simulink model "model"  (R2014a)
(part 8 of 8)

  _CN_287115458_300000_CN_287115460_300000/RConn3 -- T_287115460__/LConn3 -- bus157/LConn1
  _CN_287115458_300000_CN_355844786_300000/RConn1 -- T_355844786_300000_Hof_transformator/LConn1 -- _CN_355844786_300000_CN_51854396_300000/LConn1
  _CN_287115458_300000_CN_355844786_300000/RConn2 -- T_355844786_300000_Hof_transformator/LConn2 -- _CN_355844786_300000_CN_51854396_300000/LConn2
  _CN_287115458_300000_CN_355844786_300000/RConn3 -- T_355844786_300000_Hof_transformator/LConn3 -- _CN_355844786_300000_CN_51854396_300000/LConn3 -- bus158/LConn1
  Førre_Saurdal_CN_285935887_300000_CN_285915728_300000/RConn1 -- T_285935887__Saurdal_transformatorstasjon/RConn1 -- L_285935887/LConn1
  Førre_Saurdal_CN_285935887_300000_CN_285915728_300000/RConn2 -- T_285935887__Saurdal_transformatorstasjon/RConn2 -- L_285935887/LConn2
  Førre_Saurdal_CN_285935887_300000_CN_285915728_300000/RConn3 -- T_285935887__Saurdal_transformatorstasjon/RConn3 -- L_285935887/LConn3 -- bus159/LConn1
  _CN_355844786_300000_CN_51854396_300000/RConn1 -- T_51854396_420000;300000;132000_Tveiten/RConn1 -- _CN_206538656_300000_CN_51854396_300000/LConn1
  _CN_355844786_300000_CN_51854396_300000/RConn2 -- T_51854396_420000;300000;132000_Tveiten/RConn2 -- _CN_206538656_300000_CN_51854396_300000/LConn2
  _CN_355844786_300000_CN_51854396_300000/RConn3 -- T_51854396_420000;300000;132000_Tveiten/RConn3 -- _CN_206538656_300000_CN_51854396_300000/LConn3 -- bus160/LConn1
  Feda_Åna_Sira_CN_284275993_300000_CN_174418125_300000/LConn1 -- T_284275993_300000_/LConn1 -- Åna_Sira_Kjelland_CN_284275993_300000_CN_124861857_300000/LConn1
  Feda_Åna_Sira_CN_284275993_300000_CN_174418125_300000/LConn2 -- T_284275993_300000_/LConn2 -- Åna_Sira_Kjelland_CN_284275993_300000_CN_124861857_300000/LConn2
  Feda_Åna_Sira_CN_284275993_300000_CN_174418125_300000/LConn3 -- T_284275993_300000_/LConn3 -- Åna_Sira_Kjelland_CN_284275993_300000_CN_124861857_300000/LConn3 -- bus161/LConn1
  Feda_Åna_Sira_CN_284275993_300000_CN_174418125_300000/RConn1 -- T_174418125_300000_Feda_trafostasjon/LConn1 -- Feda_Vennesla_CN_287687994_300000_CN_174418125_300000/LConn1 -- _CN_296076234_300000_CN_174418125_300000/LConn1 -- _CN_174418125_300000_CN_174418126_300000/LConn1 -- Tonstad_Feda_CN_285825051_300000_CN_174418125_300000/RConn1
  Feda_Åna_Sira_CN_284275993_300000_CN_174418125_300000/RConn2 -- T_174418125_300000_Feda_trafostasjon/LConn2 -- Feda_Vennesla_CN_287687994_300000_CN_174418125_300000/LConn2 -- _CN_296076234_300000_CN_174418125_300000/LConn2 -- _CN_174418125_300000_CN_174418126_300000/LConn2 -- Tonstad_Feda_CN_285825051_300000_CN_174418125_300000/RConn2
  Feda_Åna_Sira_CN_284275993_300000_CN_174418125_300000/RConn3 -- T_174418125_300000_Feda_trafostasjon/LConn3 -- Feda_Vennesla_CN_287687994_300000_CN_174418125_300000/LConn3 -- _CN_296076234_300000_CN_174418125_300000/LConn3 -- _CN_174418125_300000_CN_174418126_300000/LConn3 -- bus162/LConn1 -- Tonstad_Feda_CN_285825051_300000_CN_174418125_300000/RConn3
  Åna_Sira_Kjelland_CN_284275993_300000_CN_124861857_300000/RConn1 -- T_124861857__Kjelland_transformatorstasjon/LConn1 -- Kjelland_Stokkeland_CN_124861857_300000_CN_88147266_300000/RConn1
  Åna_Sira_Kjelland_CN_284275993_300000_CN_124861857_300000/RConn2 -- T_124861857__Kjelland_transformatorstasjon/LConn2 -- Kjelland_Stokkeland_CN_124861857_300000_CN_88147266_300000/RConn2
  Åna_Sira_Kjelland_CN_284275993_300000_CN_124861857_300000/RConn3 -- T_124861857__Kjelland_transformatorstasjon/LConn3 -- Kjelland_Stokkeland_CN_124861857_300000_CN_88147266_300000/RConn3 -- bus163/LConn1
  Solhom_Tonstad_CN_285825051_300000_CN_295295263_300000/RConn1 -- T_295295263__/LConn1 -- Arendal_Solhom_CN_295295263_300000_CN_297392932_300000/LConn1
  Solhom_Tonstad_CN_285825051_300000_CN_295295263_300000/RConn2 -- T_295295263__/LConn2 -- Arendal_Solhom_CN_295295263_300000_CN_297392932_300000/LConn2
  Solhom_Tonstad_CN_285825051_300000_CN_295295263_300000/RConn3 -- T_295295263__/LConn3 -- Arendal_Solhom_CN_295295263_300000_CN_297392932_300000/LConn3 -- bus164/LConn1
  Arendal_Solhom_CN_295295263_300000_CN_297392932_300000/RConn1 -- T_297392932__Arendal_transformator/LConn1 -- Arendal_Vennesla_CN_287687994_300000_CN_297392932_300000/LConn1 -- _CN_297392932_300000_CN_358915801_300000/LConn1
  Arendal_Solhom_CN_295295263_300000_CN_297392932_300000/RConn2 -- T_297392932__Arendal_transformator/LConn2 -- Arendal_Vennesla_CN_287687994_300000_CN_297392932_300000/LConn2 -- _CN_297392932_300000_CN_358915801_300000/LConn2
  Arendal_Solhom_CN_295295263_300000_CN_297392932_300000/RConn3 -- T_297392932__Arendal_transformator/LConn3 -- Arendal_Vennesla_CN_287687994_300000_CN_297392932_300000/LConn3 -- _CN_297392932_300000_CN_358915801_300000/LConn3 -- bus165/LConn1
  Eidanger_Rød_CN_206538656_300000_CN_100648754_300000/LConn1 -- T_206538656_420000;300000;132000_Rød_transformatorstasjon/RConn1 -- _CN_206538656_300000_CN_51854396_300000/RConn1
  Eidanger_Rød_CN_206538656_300000_CN_100648754_300000/LConn2 -- T_206538656_420000;300000;132000_Rød_transformatorstasjon/RConn2 -- _CN_206538656_300000_CN_51854396_300000/RConn2
  Eidanger_Rød_CN_206538656_300000_CN_100648754_300000/LConn3 -- T_206538656_420000;300000;132000_Rød_transformatorstasjon/RConn3 -- _CN_206538656_300000_CN_51854396_300000/RConn3 -- bus166/LConn1
  Eidanger_Rød_CN_206538656_300000_CN_100648754_300000/RConn1 -- T_100648754_300000;132000_/LConn1 -- Bamble_Porsgrunn_CN_100648754_300000_CN_206628449_300000/LConn1
  Eidanger_Rød_CN_206538656_300000_CN_100648754_300000/RConn2 -- T_100648754_300000;132000_/LConn2 -- Bamble_Porsgrunn_CN_100648754_300000_CN_206628449_300000/LConn2
  Eidanger_Rød_CN_206538656_300000_CN_100648754_300000/RConn3 -- T_100648754_300000;132000_/LConn3 -- Bamble_Porsgrunn_CN_100648754_300000_CN_206628449_300000/LConn3 -- bus167/LConn1
  Rjukan_Songa_CN_288685602_300000_CN_288812256_300000/RConn1 -- T_288812256__Songa_kraftverk/LConn1 -- Kvilldal_Songa_CN_288812256_300000_CN_214181609_300000/LConn1 -- Songa_Vinje_CN_285750826_300000_CN_288812256_300000/LConn1
  Rjukan_Songa_CN_288685602_300000_CN_288812256_300000/RConn2 -- T_288812256__Songa_kraftverk/LConn2 -- Kvilldal_Songa_CN_288812256_300000_CN_214181609_300000/LConn2 -- Songa_Vinje_CN_285750826_300000_CN_288812256_300000/LConn2
  Rjukan_Songa_CN_288685602_300000_CN_288812256_300000/RConn3 -- T_288812256__Songa_kraftverk/LConn3 -- Kvilldal_Songa_CN_288812256_300000_CN_214181609_300000/LConn3 -- bus168/LConn1 -- Songa_Vinje_CN_285750826_300000_CN_288812256_300000/LConn3
  T_265770276__/LConn1 -- _CN_265770276_300000_CN_297388897_300000/LConn1
  T_265770276__/LConn2 -- _CN_265770276_300000_CN_297388897_300000/LConn2
  _CN_265770276_300000_CN_297388897_300000/LConn3 -- T_265770276__/LConn3 -- bus169/LConn1
  T_297388897_300000_Fåberg_trafostasjon/LConn1 -- _CN_265770276_300000_CN_297388897_300000/RConn1
  T_297388897_300000_Fåberg_trafostasjon/LConn2 -- _CN_265770276_300000_CN_297388897_300000/RConn2
  _CN_265770276_300000_CN_297388897_300000/RConn3 -- T_297388897_300000_Fåberg_trafostasjon/LConn3 -- bus170/LConn1
  T_290373414_300000;132000_/LConn1 -- _CN_290373414_300000_CN_290390502_300000/LConn1
  T_290373414_300000;132000_/LConn2 -- _CN_290373414_300000_CN_290390502_300000/LConn2
  _CN_290373414_300000_CN_290390502_300000/LConn3 -- T_290373414_300000;132000_/LConn3 -- bus171/LConn1
  _CN_290373414_300000_CN_290390502_300000/RConn1 -- T_290390502_300000_/LConn1 -- _CN_330825503_300000_CN_290390502_300000/LConn1
  _CN_290373414_300000_CN_290390502_300000/RConn2 -- T_290390502_300000_/LConn2 -- _CN_330825503_300000_CN_290390502_300000/LConn2
  _CN_290373414_300000_CN_290390502_300000/RConn3 -- T_290390502_300000_/LConn3 -- _CN_330825503_300000_CN_290390502_300000/LConn3 -- bus172/LConn1
  T_288810920__/LConn1 -- Nesflaten_Rjukan_CN_288810920_300000_CN_430780474_300000/LConn1
  T_288810920__/LConn2 -- Nesflaten_Rjukan_CN_288810920_300000_CN_430780474_300000/LConn2
  Nesflaten_Rjukan_CN_288810920_300000_CN_430780474_300000/LConn3 -- T_288810920__/LConn3 -- bus173/LConn1
  T_430780474__/LConn1 -- Nesflaten_Rjukan_CN_288810920_300000_CN_430780474_300000/RConn1
  T_430780474__/LConn2 -- Nesflaten_Rjukan_CN_288810920_300000_CN_430780474_300000/RConn2
  Nesflaten_Rjukan_CN_288810920_300000_CN_430780474_300000/RConn3 -- T_430780474__/LConn3 -- bus174/LConn1
  T_285750826__Vinje_kraftverk/LConn1 -- Songa_Vinje_CN_285750826_300000_CN_288812256_300000/RConn1
  T_285750826__Vinje_kraftverk/LConn2 -- Songa_Vinje_CN_285750826_300000_CN_288812256_300000/RConn2
  Songa_Vinje_CN_285750826_300000_CN_288812256_300000/RConn3 -- T_285750826__Vinje_kraftverk/LConn3 -- bus175/LConn1
  T_109810733_300000;132000_Smestad_trafostasjon/LConn1 -- _CN_46873771_300000_CN_109810733_300000/RConn1
  T_109810733_300000;132000_Smestad_trafostasjon/LConn2 -- _CN_46873771_300000_CN_109810733_300000/RConn2
  _CN_46873771_300000_CN_109810733_300000/RConn3 -- T_109810733_300000;132000_Smestad_trafostasjon/LConn3 -- bus176/LConn1
  T_229396655__/LConn1 -- _CN_229396655_300000_CN_333991713_300000/LConn1
  T_229396655__/LConn2 -- _CN_229396655_300000_CN_333991713_300000/LConn2
  _CN_229396655_300000_CN_333991713_300000/LConn3 -- T_229396655__/LConn3 -- bus177/LConn1
  _CN_229396655_300000_CN_333991713_300000/RConn1 -- T_333991713__Fana_transformatorstasjon/LConn1 -- Fana_Samnanger_CN_333991713_300000_CN_350332649_300000/LConn1 -- _CN_333991713_300000_CN_259135596_300000/LConn1
  _CN_229396655_300000_CN_333991713_300000/RConn2 -- T_333991713__Fana_transformatorstasjon/LConn2 -- Fana_Samnanger_CN_333991713_300000_CN_350332649_300000/LConn2 -- _CN_333991713_300000_CN_259135596_300000/LConn2
  _CN_229396655_300000_CN_333991713_300000/RConn3 -- T_333991713__Fana_transformatorstasjon/LConn3 -- Fana_Samnanger_CN_333991713_300000_CN_350332649_300000/LConn3 -- _CN_333991713_300000_CN_259135596_300000/LConn3 -- bus178/LConn1
  T_350332649__Samnanger/LConn1 -- Fana_Samnanger_CN_333991713_300000_CN_350332649_300000/RConn1
  T_350332649__Samnanger/LConn2 -- Fana_Samnanger_CN_333991713_300000_CN_350332649_300000/RConn2
  Fana_Samnanger_CN_333991713_300000_CN_350332649_300000/RConn3 -- T_350332649__Samnanger/LConn3 -- bus179/LConn1
  T_259135596__/LConn1 -- _CN_333991713_300000_CN_259135596_300000/RConn1
  T_259135596__/LConn2 -- _CN_333991713_300000_CN_259135596_300000/RConn2
  _CN_333991713_300000_CN_259135596_300000/RConn3 -- T_259135596__/LConn3 -- bus180/LConn1
  Bamble_Porsgrunn_CN_100648754_300000_CN_206628449_300000/RConn1 -- T_206628449__Bamble/RConn1 -- L_206628449/LConn1
  Bamble_Porsgrunn_CN_100648754_300000_CN_206628449_300000/RConn2 -- T_206628449__Bamble/RConn2 -- L_206628449/LConn2
  Bamble_Porsgrunn_CN_100648754_300000_CN_206628449_300000/RConn3 -- T_206628449__Bamble/RConn3 -- L_206628449/LConn3 -- bus181/LConn1
  T_114336709_300000;132000_Vang_trafostasjon/LConn1 -- Minne_Brenneriroa_CN_120279477_300000_CN_114336709_300000/RConn1
  T_114336709_300000;132000_Vang_trafostasjon/LConn2 -- Minne_Brenneriroa_CN_120279477_300000_CN_114336709_300000/RConn2
  Minne_Brenneriroa_CN_120279477_300000_CN_114336709_300000/RConn3 -- T_114336709_300000;132000_Vang_trafostasjon/LConn3 -- bus182/LConn1
  Førre_Hylen_CN_285915728_300000_CN_289304147_300000/RConn1 -- T_289304147__/LConn1 -- Sauda_Hylen_CN_289304147_300000_CN_285805418_300000/RConn1
  Førre_Hylen_CN_285915728_300000_CN_289304147_300000/RConn2 -- T_289304147__/LConn2 -- Sauda_Hylen_CN_289304147_300000_CN_285805418_300000/RConn2
  Førre_Hylen_CN_285915728_300000_CN_289304147_300000/RConn3 -- T_289304147__/LConn3 -- Sauda_Hylen_CN_289304147_300000_CN_285805418_300000/RConn3 -- bus183/LConn1
  Arendal_Vennesla_CN_287687994_300000_CN_297392932_300000/RConn1 -- T_287687994_420000;300000_/RConn1 -- Feda_Vennesla_CN_287687994_300000_CN_174418125_300000/RConn1
  Arendal_Vennesla_CN_287687994_300000_CN_297392932_300000/RConn2 -- T_287687994_420000;300000_/RConn2 -- Feda_Vennesla_CN_287687994_300000_CN_174418125_300000/RConn2
  Arendal_Vennesla_CN_287687994_300000_CN_297392932_300000/RConn3 -- T_287687994_420000;300000_/RConn3 -- Feda_Vennesla_CN_287687994_300000_CN_174418125_300000/RConn3 -- bus184/LConn1
  T_330825503_300000;132000_/LConn1 -- _CN_330825503_300000_CN_290390502_300000/RConn1
  T_330825503_300000;132000_/LConn2 -- _CN_330825503_300000_CN_290390502_300000/RConn2
  _CN_330825503_300000_CN_290390502_300000/RConn3 -- T_330825503_300000;132000_/LConn3 -- bus185/LConn1
  _CN_296076234_300000_CN_296076235_300000/LConn1 -- T_296076234_300000_/LConn1 -- _CN_296076234_300000_CN_174418125_300000/RConn1
  _CN_296076234_300000_CN_296076235_300000/LConn2 -- T_296076234_300000_/LConn2 -- _CN_296076234_300000_CN_174418125_300000/RConn2
  _CN_296076234_300000_CN_296076235_300000/LConn3 -- T_296076234_300000_/LConn3 -- _CN_296076234_300000_CN_174418125_300000/RConn3 -- bus186/LConn1
  T_296076235_300000;132000_/LConn1 -- _CN_296076234_300000_CN_296076235_300000/RConn1
  T_296076235_300000;132000_/LConn2 -- _CN_296076234_300000_CN_296076235_300000/RConn2
  _CN_296076234_300000_CN_296076235_300000/RConn3 -- T_296076235_300000;132000_/LConn3 -- bus187/LConn1
  T_174418126_300000_Feda_static_inverter_plant/LConn1 -- _CN_174418125_300000_CN_174418126_300000/RConn1
  T_174418126_300000_Feda_static_inverter_plant/LConn2 -- _CN_174418125_300000_CN_174418126_300000/RConn2
  _CN_174418125_300000_CN_174418126_300000/RConn3 -- T_174418126_300000_Feda_static_inverter_plant/LConn3 -- bus188/LConn1
  T_400655825_300000;132000_/LConn1 -- _CN_400655825_300000_CN_201483501_300000/LConn1
  T_400655825_300000;132000_/LConn2 -- _CN_400655825_300000_CN_201483501_300000/LConn2
  _CN_400655825_300000_CN_201483501_300000/LConn3 -- T_400655825_300000;132000_/LConn3 -- bus189/LConn1
  _CN_400655825_300000_CN_201483501_300000/RConn1 -- T_201483501_420000;300000;132000_/RConn1 -- L_201483501/LConn1
  _CN_400655825_300000_CN_201483501_300000/RConn2 -- T_201483501_420000;300000;132000_/RConn2 -- L_201483501/LConn2
  _CN_400655825_300000_CN_201483501_300000/RConn3 -- T_201483501_420000;300000;132000_/RConn3 -- L_201483501/LConn3 -- bus190/LConn1
  T_289304185__/LConn1 -- _CN_289304185_300000_CN_285805418_300000/RConn1
  T_289304185__/LConn2 -- _CN_289304185_300000_CN_285805418_300000/RConn2
  _CN_289304185_300000_CN_285805418_300000/RConn3 -- T_289304185__/LConn3 -- bus191/LConn1
  _CN_297392932_300000_CN_358915801_300000/RConn1 -- T_358915801_420000_/RConn1 -- L_358915801/LConn1
  _CN_297392932_300000_CN_358915801_300000/RConn2 -- T_358915801_420000_/RConn2 -- L_358915801/LConn2
  _CN_297392932_300000_CN_358915801_300000/RConn3 -- T_358915801_420000_/RConn3 -- L_358915801/LConn3 -- bus192/LConn1
  G_71356608_Roskrepp_kraftverk/RConn1 -- Roskrepp_Duge_CN_261717967_300000_CN_71356608_300000/RConn1
  G_71356608_Roskrepp_kraftverk/RConn2 -- Roskrepp_Duge_CN_261717967_300000_CN_71356608_300000/RConn2
  Roskrepp_Duge_CN_261717967_300000_CN_71356608_300000/RConn3 -- G_71356608_Roskrepp_kraftverk/RConn3 -- bus193/LConn1
  Kvilldal_Songa_CN_288812256_300000_CN_214181609_300000/RConn1 -- T_214181609__/RConn1 -- L_214181609/LConn1
  Kvilldal_Songa_CN_288812256_300000_CN_214181609_300000/RConn2 -- T_214181609__/RConn2 -- L_214181609/LConn2
  Kvilldal_Songa_CN_288812256_300000_CN_214181609_300000/RConn3 -- T_214181609__/RConn3 -- L_214181609/LConn3 -- bus194/LConn1
  T_353884513__/LConn1 -- Røldal_Tyssedal_CN_353884513_300000_CN_242396005_300000/LConn1
  T_353884513__/LConn2 -- Røldal_Tyssedal_CN_353884513_300000_CN_242396005_300000/LConn2
  Røldal_Tyssedal_CN_353884513_300000_CN_242396005_300000/LConn3 -- T_353884513__/LConn3 -- bus195/LConn1
  T_242396005__/LConn1 -- Røldal_Tyssedal_CN_353884513_300000_CN_242396005_300000/RConn1
  T_242396005__/LConn2 -- Røldal_Tyssedal_CN_353884513_300000_CN_242396005_300000/RConn2
  Røldal_Tyssedal_CN_353884513_300000_CN_242396005_300000/RConn3 -- T_242396005__/LConn3 -- bus196/LConn1
  T_254428135_300000_/LConn1 -- _CN_254428135_300000_CN_229806969_300000/LConn1
  T_254428135_300000_/LConn2 -- _CN_254428135_300000_CN_229806969_300000/LConn2
  _CN_254428135_300000_CN_229806969_300000/LConn3 -- T_254428135_300000_/LConn3 -- bus197/LConn1
  _CN_254428135_300000_CN_229806969_300000/RConn1 -- T_229806969_300000_/LConn1 -- _CN_229806969_300000_CN_229806970_300000/LConn1
  _CN_254428135_300000_CN_229806969_300000/RConn2 -- T_229806969_300000_/LConn2 -- _CN_229806969_300000_CN_229806970_300000/LConn2
  _CN_254428135_300000_CN_229806969_300000/RConn3 -- T_229806969_300000_/LConn3 -- _CN_229806969_300000_CN_229806970_300000/LConn3 -- bus198/LConn1
  T_229806970__/LConn1 -- _CN_229806969_300000_CN_229806970_300000/RConn1
  T_229806970__/LConn2 -- _CN_229806969_300000_CN_229806970_300000/RConn2
  _CN_229806969_300000_CN_229806970_300000/RConn3 -- T_229806970__/LConn3 -- bus199/LConn1
  T_202200066_420000;132000_Viklandet/LConn1 -- _CN_202200066_420000_CN_290393697_420000/LConn1
  T_202200066_420000;132000_Viklandet/LConn2 -- _CN_202200066_420000_CN_290393697_420000/LConn2
  _CN_202200066_420000_CN_290393697_420000/LConn3 -- T_202200066_420000;132000_Viklandet/LConn3 -- bus200/LConn1
  T_290393697_420000;300000_Aura/LConn1 -- _CN_202200066_420000_CN_290393697_420000/RConn1
  T_290393697_420000;300000_Aura/LConn2 -- _CN_202200066_420000_CN_290393697_420000/RConn2
  _CN_202200066_420000_CN_290393697_420000/RConn3 -- T_290393697_420000;300000_Aura/LConn3 -- bus201/LConn1
  T_114318083__/LConn1 -- _CN_114318083_420000_CN_114318078_420000/LConn1
  T_114318083__/LConn2 -- _CN_114318083_420000_CN_114318078_420000/LConn2
  _CN_114318083_420000_CN_114318078_420000/LConn3 -- T_114318083__/LConn3 -- bus202/LConn1
  _CN_114318083_420000_CN_114318078_420000/RConn1 -- T_114318078__/LConn1 -- _CN_29578389_420000_CN_114318078_420000/LConn1
  _CN_114318083_420000_CN_114318078_420000/RConn2 -- T_114318078__/LConn2 -- _CN_29578389_420000_CN_114318078_420000/LConn2
  _CN_114318083_420000_CN_114318078_420000/RConn3 -- T_114318078__/LConn3 -- _CN_29578389_420000_CN_114318078_420000/LConn3 -- bus203/LConn1
  T_232893576_420000_Halden/LConn1 -- Halden_Hasle_CN_232893576_420000_CN_60495669_420000/LConn1
  T_232893576_420000_Halden/LConn2 -- Halden_Hasle_CN_232893576_420000_CN_60495669_420000/LConn2
  Halden_Hasle_CN_232893576_420000_CN_60495669_420000/LConn3 -- T_232893576_420000_Halden/LConn3 -- bus204/LConn1
  Halden_Hasle_CN_232893576_420000_CN_60495669_420000/RConn1 -- T_60495669_420000;300000;132000_Hasle_Transformatorstasjon/LConn1 -- Hasle_Rød_CN_51856017_420000_CN_60495669_420000/LConn1 -- _CN_29578389_420000_CN_60495669_420000/LConn1
  Halden_Hasle_CN_232893576_420000_CN_60495669_420000/RConn2 -- T_60495669_420000;300000;132000_Hasle_Transformatorstasjon/LConn2 -- Hasle_Rød_CN_51856017_420000_CN_60495669_420000/LConn2 -- _CN_29578389_420000_CN_60495669_420000/LConn2
  Halden_Hasle_CN_232893576_420000_CN_60495669_420000/RConn3 -- T_60495669_420000;300000;132000_Hasle_Transformatorstasjon/LConn3 -- Hasle_Rød_CN_51856017_420000_CN_60495669_420000/LConn3 -- _CN_29578389_420000_CN_60495669_420000/LConn3 -- bus205/LConn1
  T_285935887__Saurdal_transformatorstasjon/LConn1 -- Kvilldal_Saurdal_CN_285935887_420000_CN_214181609_420000/LConn1
  T_285935887__Saurdal_transformatorstasjon/LConn2 -- Kvilldal_Saurdal_CN_285935887_420000_CN_214181609_420000/LConn2
  Kvilldal_Saurdal_CN_285935887_420000_CN_214181609_420000/LConn3 -- T_285935887__Saurdal_transformatorstasjon/LConn3 -- bus206/LConn1
  T_214181609__/LConn1 -- Kvilldal_Saurdal_CN_285935887_420000_CN_214181609_420000/RConn1
  T_214181609__/LConn2 -- Kvilldal_Saurdal_CN_285935887_420000_CN_214181609_420000/RConn2
  Kvilldal_Saurdal_CN_285935887_420000_CN_214181609_420000/RConn3 -- T_214181609__/LConn3 -- bus207/LConn1
  Hasle_Rød_CN_51856017_420000_CN_51855380_420000/LConn1 -- T_51856017__/LConn1 -- Hasle_Rød_CN_51856017_420000_CN_60495669_420000/RConn1
  Hasle_Rød_CN_51856017_420000_CN_51855380_420000/LConn2 -- T_51856017__/LConn2 -- Hasle_Rød_CN_51856017_420000_CN_60495669_420000/RConn2
  Hasle_Rød_CN_51856017_420000_CN_51855380_420000/LConn3 -- T_51856017__/LConn3 -- Hasle_Rød_CN_51856017_420000_CN_60495669_420000/RConn3 -- bus208/LConn1
  Hasle_Rød_CN_51856017_420000_CN_51855380_420000/RConn1 -- T_51855380__/LConn1 -- Hasle_Rød_CN_51855380_420000_CN_51854396_420000/LConn1
  Hasle_Rød_CN_51856017_420000_CN_51855380_420000/RConn2 -- T_51855380__/LConn2 -- Hasle_Rød_CN_51855380_420000_CN_51854396_420000/LConn2
  Hasle_Rød_CN_51856017_420000_CN_51855380_420000/RConn3 -- T_51855380__/LConn3 -- Hasle_Rød_CN_51855380_420000_CN_51854396_420000/LConn3 -- bus209/LConn1
  T_295444099_420000;300000;66000_Frogner_transformatorstasjon/LConn1 -- _CN_295444099_420000_CN_100151486_420000/LConn1
  T_295444099_420000;300000;66000_Frogner_transformatorstasjon/LConn2 -- _CN_295444099_420000_CN_100151486_420000/LConn2
  _CN_295444099_420000_CN_100151486_420000/LConn3 -- T_295444099_420000;300000;66000_Frogner_transformatorstasjon/LConn3 -- bus210/LConn1
  _CN_295444099_420000_CN_100151486_420000/RConn1 -- T_100151486_420000_Ski/LConn1 -- _CN_29578389_420000_CN_100151486_420000/LConn1
  _CN_295444099_420000_CN_100151486_420000/RConn2 -- T_100151486_420000_Ski/LConn2 -- _CN_29578389_420000_CN_100151486_420000/LConn2
  _CN_295444099_420000_CN_100151486_420000/RConn3 -- T_100151486_420000_Ski/LConn3 -- _CN_29578389_420000_CN_100151486_420000/LConn3 -- bus211/LConn1
  Hasle_Rød_CN_51855380_420000_CN_51854396_420000/RConn1 -- T_51854396_420000;300000;132000_Tveiten/LConn1 -- Hasle_Rød_CN_206538656_420000_CN_51854396_420000/LConn1
  Hasle_Rød_CN_51855380_420000_CN_51854396_420000/RConn2 -- T_51854396_420000;300000;132000_Tveiten/LConn2 -- Hasle_Rød_CN_206538656_420000_CN_51854396_420000/LConn2
  Hasle_Rød_CN_51855380_420000_CN_51854396_420000/RConn3 -- T_51854396_420000;300000;132000_Tveiten/LConn3 -- Hasle_Rød_CN_206538656_420000_CN_51854396_420000/LConn3 -- bus212/LConn1
  _CN_29578389_420000_CN_60495669_420000/RConn1 -- T_29578389_420000_/LConn1 -- _CN_29578389_420000_CN_114318078_420000/RConn1 -- _CN_29578389_420000_CN_100151486_420000/RConn1
  _CN_29578389_420000_CN_60495669_420000/RConn2 -- T_29578389_420000_/LConn2 -- _CN_29578389_420000_CN_114318078_420000/RConn2 -- _CN_29578389_420000_CN_100151486_420000/RConn2
  _CN_29578389_420000_CN_60495669_420000/RConn3 -- T_29578389_420000_/LConn3 -- _CN_29578389_420000_CN_114318078_420000/RConn3 -- _CN_29578389_420000_CN_100151486_420000/RConn3 -- bus213/LConn1
  Bamble_Rød_CN_206538656_420000_CN_206628453_420000/LConn1 -- T_206538656_420000;300000;132000_Rød_transformatorstasjon/LConn1 -- Hasle_Rød_CN_206538656_420000_CN_51854396_420000/RConn1
  Bamble_Rød_CN_206538656_420000_CN_206628453_420000/LConn2 -- T_206538656_420000;300000;132000_Rød_transformatorstasjon/LConn2 -- Hasle_Rød_CN_206538656_420000_CN_51854396_420000/RConn2
  Bamble_Rød_CN_206538656_420000_CN_206628453_420000/LConn3 -- T_206538656_420000;300000;132000_Rød_transformatorstasjon/LConn3 -- Hasle_Rød_CN_206538656_420000_CN_51854396_420000/RConn3 -- bus214/LConn1
  Bamble_Rød_CN_206538656_420000_CN_206628453_420000/RConn1 -- T_206628453__Grenland/LConn1 -- Bamble_Rød_CN_206628449_420000_CN_206628453_420000/LConn1
  Bamble_Rød_CN_206538656_420000_CN_206628453_420000/RConn2 -- T_206628453__Grenland/LConn2 -- Bamble_Rød_CN_206628449_420000_CN_206628453_420000/LConn2
  Bamble_Rød_CN_206538656_420000_CN_206628453_420000/RConn3 -- T_206628453__Grenland/LConn3 -- Bamble_Rød_CN_206628449_420000_CN_206628453_420000/LConn3 -- bus215/LConn1
  T_296238635__/LConn1 -- Hol_Dagali(?)_CN_296238635_420000_CN_296229069_420000/LConn1
  T_296238635__/LConn2 -- Hol_Dagali(?)_CN_296238635_420000_CN_296229069_420000/LConn2
  Hol_Dagali(?)_CN_296238635_420000_CN_296229069_420000/LConn3 -- T_296238635__/LConn3 -- bus216/LConn1
  T_296229069__/LConn1 -- Hol_Dagali(?)_CN_296238635_420000_CN_296229069_420000/RConn1
  T_296229069__/LConn2 -- Hol_Dagali(?)_CN_296238635_420000_CN_296229069_420000/RConn2
  Hol_Dagali(?)_CN_296238635_420000_CN_296229069_420000/RConn3 -- T_296229069__/LConn3 -- bus217/LConn1
  T_287687994_420000;300000_/LConn1 -- Tokke_Vennesla_CN_287687994_420000_CN_244179408_420000/LConn1
  T_287687994_420000;300000_/LConn2 -- Tokke_Vennesla_CN_287687994_420000_CN_244179408_420000/LConn2
  Tokke_Vennesla_CN_287687994_420000_CN_244179408_420000/LConn3 -- T_287687994_420000;300000_/LConn3 -- bus218/LConn1
  G_244179408_Brokke_Kraftverk/RConn1 -- Tokke_Vennesla_CN_287687994_420000_CN_244179408_420000/RConn1
  G_244179408_Brokke_Kraftverk/RConn2 -- Tokke_Vennesla_CN_287687994_420000_CN_244179408_420000/RConn2
  Tokke_Vennesla_CN_287687994_420000_CN_244179408_420000/RConn3 -- G_244179408_Brokke_Kraftverk/RConn3 -- bus219/LConn1
  T_197866182_420000;132000_/LConn1 -- _CN_197866182_420000_CN_201483501_420000/LConn1
  T_197866182_420000;132000_/LConn2 -- _CN_197866182_420000_CN_201483501_420000/LConn2
  _CN_197866182_420000_CN_201483501_420000/LConn3 -- T_197866182_420000;132000_/LConn3 -- bus220/LConn1
  T_201483501_420000;300000;132000_/LConn1 -- _CN_197866182_420000_CN_201483501_420000/RConn1
  T_201483501_420000;300000;132000_/LConn2 -- _CN_197866182_420000_CN_201483501_420000/RConn2
  _CN_197866182_420000_CN_201483501_420000/RConn3 -- T_201483501_420000;300000;132000_/LConn3 -- bus221/LConn1
  T_205115991_420000;132000_Ringerike_trafostasjon/LConn1 -- _CN_205115991_420000_CN_295444089_420000/LConn1
  T_205115991_420000;132000_Ringerike_trafostasjon/LConn2 -- _CN_205115991_420000_CN_295444089_420000/LConn2
  _CN_205115991_420000_CN_295444089_420000/LConn3 -- T_205115991_420000;132000_Ringerike_trafostasjon/LConn3 -- bus222/LConn1
  T_295444089_420000_Ådal_trafostasjon/LConn1 -- _CN_205115991_420000_CN_295444089_420000/RConn1
  T_295444089_420000_Ådal_trafostasjon/LConn2 -- _CN_205115991_420000_CN_295444089_420000/RConn2
  _CN_205115991_420000_CN_295444089_420000/RConn3 -- T_295444089_420000_Ådal_trafostasjon/LConn3 -- bus223/LConn1
  T_358915801_420000_/LConn1 -- Arendal_Bamble_CN_358915801_420000_CN_206628449_420000/LConn1
  T_358915801_420000_/LConn2 -- Arendal_Bamble_CN_358915801_420000_CN_206628449_420000/LConn2
  Arendal_Bamble_CN_358915801_420000_CN_206628449_420000/LConn3 -- T_358915801_420000_/LConn3 -- bus224/LConn1
  Arendal_Bamble_CN_358915801_420000_CN_206628449_420000/RConn1 -- T_206628449__Bamble/LConn1 -- Bamble_Rød_CN_206628449_420000_CN_206628453_420000/RConn1
  Arendal_Bamble_CN_358915801_420000_CN_206628449_420000/RConn2 -- T_206628449__Bamble/LConn2 -- Bamble_Rød_CN_206628449_420000_CN_206628453_420000/RConn2
  Arendal_Bamble_CN_358915801_420000_CN_206628449_420000/RConn3 -- T_206628449__Bamble/LConn3 -- Bamble_Rød_CN_206628449_420000_CN_206628453_420000/RConn3 -- bus225/LConn1
  T_287685850_420000;300000_/LConn1 -- _CN_287685850_420000_CN_287684722_420000/LConn1
  T_287685850_420000;300000_/LConn2 -- _CN_287685850_420000_CN_287684722_420000/LConn2
  _CN_287685850_420000_CN_287684722_420000/LConn3 -- T_287685850_420000;300000_/LConn3 -- bus226/LConn1
  T_287684722_420000_/LConn1 -- _CN_287685850_420000_CN_287684722_420000/RConn1
  T_287684722_420000_/LConn2 -- _CN_287685850_420000_CN_287684722_420000/RConn2
  _CN_287685850_420000_CN_287684722_420000/RConn3 -- T_287684722_420000_/LConn3 -- bus227/LConn1
  T_288861057__Sande_transformatorstasjon/RConn1 -- L_288861057/LConn1
  T_288861057__Sande_transformatorstasjon/RConn2 -- L_288861057/LConn2
  L_288861057/LConn3 -- T_288861057__Sande_transformatorstasjon/RConn3 -- bus228/LConn1
  T_75805059__Forus_transformatorstasjon/RConn1 -- L_75805059/LConn1
  T_75805059__Forus_transformatorstasjon/RConn2 -- L_75805059/LConn2
  L_75805059/LConn3 -- T_75805059__Forus_transformatorstasjon/RConn3 -- bus229/LConn1
  T_41226817_50000;10000_Jåttå_transformatorstasjon/RConn1 -- L_41226817/LConn1
  T_41226817_50000;10000_Jåttå_transformatorstasjon/RConn2 -- L_41226817/LConn2
  L_41226817/LConn3 -- T_41226817_50000;10000_Jåttå_transformatorstasjon/RConn3 -- bus230/LConn1
  T_286505477_50000_Alsteinsgata_transformatorstasjon/RConn1 -- L_286505477/LConn1
  T_286505477_50000_Alsteinsgata_transformatorstasjon/RConn2 -- L_286505477/LConn2
  L_286505477/LConn3 -- T_286505477_50000_Alsteinsgata_transformatorstasjon/RConn3 -- bus231/LConn1
  T_296504285__Kongsgata/RConn1 -- L_296504285/LConn1
  T_296504285__Kongsgata/RConn2 -- L_296504285/LConn2
  L_296504285/LConn3 -- T_296504285__Kongsgata/RConn3 -- bus232/LConn1
  T_240212685_50000_Lura_transformatorstasjon/RConn1 -- L_240212685/LConn1
  T_240212685_50000_Lura_transformatorstasjon/RConn2 -- L_240212685/LConn2
  L_240212685/LConn3 -- T_240212685_50000_Lura_transformatorstasjon/RConn3 -- bus233/LConn1
  T_284260110_50000;22000_Opstad_trafostasjon/RConn1 -- L_284260110/LConn1
  T_284260110_50000;22000_Opstad_trafostasjon/RConn2 -- L_284260110/LConn2
  L_284260110/LConn3 -- T_284260110_50000;22000_Opstad_trafostasjon/RConn3 -- bus234/LConn1
  T_329581844_50000;medium_Nærbø_transformatorstasjon/RConn1 -- L_329581844/LConn1
  T_329581844_50000;medium_Nærbø_transformatorstasjon/RConn2 -- L_329581844/LConn2
  L_329581844/LConn3 -- T_329581844_50000;medium_Nærbø_transformatorstasjon/RConn3 -- bus235/LConn1
  T_290983494__/RConn1 -- L_290983494/LConn1
  T_290983494__/RConn2 -- L_290983494/LConn2
  L_290983494/LConn3 -- T_290983494__/RConn3 -- bus236/LConn1
  T_329581840__Kalberg_transformatorstasjon/RConn1 -- L_329581840/LConn1
  T_329581840__Kalberg_transformatorstasjon/RConn2 -- L_329581840/LConn2
  L_329581840/LConn3 -- T_329581840__Kalberg_transformatorstasjon/RConn3 -- bus237/LConn1
  T_284251750__Vagle_transformatorstasjon/RConn1 -- L_284251750/LConn1
  T_284251750__Vagle_transformatorstasjon/RConn2 -- L_284251750/LConn2
  L_284251750/LConn3 -- T_284251750__Vagle_transformatorstasjon/RConn3 -- bus238/LConn1
  T_285809906__Håland_trafostasjon/RConn1 -- L_285809906/LConn1
  T_285809906__Håland_trafostasjon/RConn2 -- L_285809906/LConn2
  L_285809906/LConn3 -- T_285809906__Håland_trafostasjon/RConn3 -- bus239/LConn1
  T_89032743__Hillevåg_transformatorstasjon/RConn1 -- L_89032743/LConn1
  T_89032743__Hillevåg_transformatorstasjon/RConn2 -- L_89032743/LConn2
  L_89032743/LConn3 -- T_89032743__Hillevåg_transformatorstasjon/RConn3 -- bus240/LConn1
  T_41226815__Ullandhaug_transformatorstasjon/RConn1 -- L_41226815/LConn1
  T_41226815__Ullandhaug_transformatorstasjon/RConn2 -- L_41226815/LConn2
  L_41226815/LConn3 -- T_41226815__Ullandhaug_transformatorstasjon/RConn3 -- bus241/LConn1
  T_112412584__Vatne_transformatorstasjon/RConn1 -- L_112412584/LConn1
  T_112412584__Vatne_transformatorstasjon/RConn2 -- L_112412584/LConn2
  L_112412584/LConn3 -- T_112412584__Vatne_transformatorstasjon/RConn3 -- bus242/LConn1
  T_329592517_50000;medium_Riska_transformatorstasjon/RConn1 -- L_329592517/LConn1
  T_329592517_50000;medium_Riska_transformatorstasjon/RConn2 -- L_329592517/LConn2
  L_329592517/LConn3 -- T_329592517_50000;medium_Riska_transformatorstasjon/RConn3 -- bus243/LConn1
  T_295444551__Buøy_transformatorstasjon/RConn1 -- L_295444551/LConn1
  T_295444551__Buøy_transformatorstasjon/RConn2 -- L_295444551/LConn2
  L_295444551/LConn3 -- T_295444551__Buøy_transformatorstasjon/RConn3 -- bus244/LConn1
  T_139346918_50000_Dusavik/RConn1 -- L_139346918/LConn1
  T_139346918_50000_Dusavik/RConn2 -- L_139346918/LConn2
  L_139346918/LConn3 -- T_139346918_50000_Dusavik/RConn3 -- bus245/LConn1
  T_289487098__Haugesundsgata_transformatorstasjon/RConn1 -- L_289487098/LConn1
  T_289487098__Haugesundsgata_transformatorstasjon/RConn2 -- L_289487098/LConn2
  L_289487098/LConn3 -- T_289487098__Haugesundsgata_transformatorstasjon/RConn3 -- bus246/LConn1
  T_91655624__/RConn1 -- L_91655624/LConn1
  T_91655624__/RConn2 -- L_91655624/LConn2
  L_91655624/LConn3 -- T_91655624__/RConn3 -- bus247/LConn1
  T_96439090__/RConn1 -- L_96439090/LConn1
  T_96439090__/RConn2 -- L_96439090/LConn2
  L_96439090/LConn3 -- T_96439090__/RConn3 -- bus248/LConn1
  T_36163257__/RConn1 -- L_36163257/LConn1
  T_36163257__/RConn2 -- L_36163257/LConn2
  L_36163257/LConn3 -- T_36163257__/RConn3 -- bus249/LConn1
  T_129017290__/RConn1 -- L_129017290/LConn1
  T_129017290__/RConn2 -- L_129017290/LConn2
  L_129017290/LConn3 -- T_129017290__/RConn3 -- bus250/LConn1
  T_297123048_50000_Båtstad_transformatorstasjon/RConn1 -- L_297123048/LConn1
  T_297123048_50000_Båtstad_transformatorstasjon/RConn2 -- L_297123048/LConn2
  L_297123048/LConn3 -- T_297123048_50000_Båtstad_transformatorstasjon/RConn3 -- bus251/LConn1
  T_297122914__Ålgård_transformatorstasjon/RConn1 -- L_297122914/LConn1
  T_297122914__Ålgård_transformatorstasjon/RConn2 -- L_297122914/LConn2
  L_297122914/LConn3 -- T_297122914__Ålgård_transformatorstasjon/RConn3 -- bus252/LConn1
  T_285976807__Tu_trafostasjon/RConn1 -- L_285976807/LConn1
  T_285976807__Tu_trafostasjon/RConn2 -- L_285976807/LConn2
  L_285976807/LConn3 -- T_285976807__Tu_trafostasjon/RConn3 -- bus253/LConn1
  T_285809905__Hatteland_trafostasjon/RConn1 -- L_285809905/LConn1
  T_285809905__Hatteland_trafostasjon/RConn2 -- L_285809905/LConn2
  L_285809905/LConn3 -- T_285809905__Hatteland_trafostasjon/RConn3 -- bus254/LConn1
  T_290896873__Kleppemarka_trafostasjon/RConn1 -- L_290896873/LConn1
  T_290896873__Kleppemarka_trafostasjon/RConn2 -- L_290896873/LConn2
  L_290896873/LConn3 -- T_290896873__Kleppemarka_trafostasjon/RConn3 -- bus255/LConn1
  T_384765294__/RConn1 -- L_384765294/LConn1
  T_384765294__/RConn2 -- L_384765294/LConn2
  L_384765294/LConn3 -- T_384765294__/RConn3 -- bus256/LConn1
  T_118272324_66000_Nerdrum_transformator/RConn1 -- L_118272324/LConn1
  T_118272324_66000_Nerdrum_transformator/RConn2 -- L_118272324/LConn2
  L_118272324/LConn3 -- T_118272324_66000_Nerdrum_transformator/RConn3 -- bus257/LConn1
  T_88729162_66000_?_transformatorstasjon/RConn1 -- L_88729162/LConn1
  T_88729162_66000_?_transformatorstasjon/RConn2 -- L_88729162/LConn2
  L_88729162/LConn3 -- T_88729162_66000_?_transformatorstasjon/RConn3 -- bus258/LConn1
  T_295444119__Vestbygata_transformatorstasjon/RConn1 -- L_295444119/LConn1
  T_295444119__Vestbygata_transformatorstasjon/RConn2 -- L_295444119/LConn2
  L_295444119/LConn3 -- T_295444119__Vestbygata_transformatorstasjon/RConn3 -- bus259/LConn1
  T_92116523__Strøm_transformatorstasjon/RConn1 -- L_92116523/LConn1
  T_92116523__Strøm_transformatorstasjon/RConn2 -- L_92116523/LConn2
  L_92116523/LConn3 -- T_92116523__Strøm_transformatorstasjon/RConn3 -- bus260/LConn1
  T_295444109__Gjestad_transformatorstasjon/RConn1 -- L_295444109/LConn1
  T_295444109__Gjestad_transformatorstasjon/RConn2 -- L_295444109/LConn2
  L_295444109/LConn3 -- T_295444109__Gjestad_transformatorstasjon/RConn3 -- bus261/LConn1
  T_98937735__/RConn1 -- L_98937735/LConn1
  T_98937735__/RConn2 -- L_98937735/LConn2
  L_98937735/LConn3 -- T_98937735__/RConn3 -- bus262/LConn1
  T_185427154__/RConn1 -- L_185427154/LConn1
  T_185427154__/RConn2 -- L_185427154/LConn2
  L_185427154/LConn3 -- T_185427154__/RConn3 -- bus263/LConn1
  T_384765297__Løken_transformator/RConn1 -- L_384765297/LConn1
  T_384765297__Løken_transformator/RConn2 -- L_384765297/LConn2
  L_384765297/LConn3 -- T_384765297__Løken_transformator/RConn3 -- bus264/LConn1
  T_90078235__/RConn1 -- L_90078235/LConn1
  T_90078235__/RConn2 -- L_90078235/LConn2
  L_90078235/LConn3 -- T_90078235__/RConn3 -- bus265/LConn1
  T_113574844__/RConn1 -- L_113574844/LConn1
  T_113574844__/RConn2 -- L_113574844/LConn2
  L_113574844/LConn3 -- T_113574844__/RConn3 -- bus266/LConn1
  T_90139980__/RConn1 -- L_90139980/LConn1
  T_90139980__/RConn2 -- L_90139980/LConn2
  L_90139980/LConn3 -- T_90139980__/RConn3 -- bus267/LConn1
  T_106879472__/RConn1 -- L_106879472/LConn1
  T_106879472__/RConn2 -- L_106879472/LConn2
  L_106879472/LConn3 -- T_106879472__/RConn3 -- bus268/LConn1
  T_202200064_132000_Aura/RConn1 -- L_202200064/LConn1
  T_202200064_132000_Aura/RConn2 -- L_202200064/LConn2
  L_202200064/LConn3 -- T_202200064_132000_Aura/RConn3 -- bus269/LConn1
  T_202200068_132000_/RConn1 -- L_202200068/LConn1
  T_202200068_132000_/RConn2 -- L_202200068/LConn2
  L_202200068/LConn3 -- T_202200068_132000_/RConn3 -- bus270/LConn1
  T_432917507__/RConn1 -- L_432917507/LConn1
  T_432917507__/RConn2 -- L_432917507/LConn2
  L_432917507/LConn3 -- T_432917507__/RConn3 -- bus271/LConn1
  T_92630533_132000_/RConn1 -- L_92630533/LConn1
  T_92630533_132000_/RConn2 -- L_92630533/LConn2
  L_92630533/LConn3 -- T_92630533_132000_/RConn3 -- bus272/LConn1
  T_26938543_132000_/RConn1 -- L_26938543/LConn1
  T_26938543_132000_/RConn2 -- L_26938543/LConn2
  L_26938543/LConn3 -- T_26938543_132000_/RConn3 -- bus273/LConn1
  T_27030901_132000_/RConn1 -- L_27030901/LConn1
  T_27030901_132000_/RConn2 -- L_27030901/LConn2
  L_27030901/LConn3 -- T_27030901_132000_/RConn3 -- bus274/LConn1
  T_355844785__/RConn1 -- L_355844785/LConn1
  T_355844785__/RConn2 -- L_355844785/LConn2
  L_355844785/LConn3 -- T_355844785__/RConn3 -- bus275/LConn1
  T_355844774__/RConn1 -- L_355844774/LConn1
  T_355844774__/RConn2 -- L_355844774/LConn2
  L_355844774/LConn3 -- T_355844774__/RConn3 -- bus276/LConn1
  T_111859753__/RConn1 -- L_111859753/LConn1
  T_111859753__/RConn2 -- L_111859753/LConn2
  L_111859753/LConn3 -- T_111859753__/RConn3 -- bus277/LConn1
  T_103088765_132000_/RConn1 -- L_103088765/LConn1
  T_103088765_132000_/RConn2 -- L_103088765/LConn2
  L_103088765/LConn3 -- T_103088765_132000_/RConn3 -- bus278/LConn1
  T_285928490_132000_/RConn1 -- L_285928490/LConn1
  T_285928490_132000_/RConn2 -- L_285928490/LConn2
  L_285928490/LConn3 -- T_285928490_132000_/RConn3 -- bus279/LConn1
  T_289829880__/RConn1 -- L_289829880/LConn1
  T_289829880__/RConn2 -- L_289829880/LConn2
  L_289829880/LConn3 -- T_289829880__/RConn3 -- bus280/LConn1
  T_331597523_132000_/RConn1 -- L_331597523/LConn1
  T_331597523_132000_/RConn2 -- L_331597523/LConn2
  L_331597523/LConn3 -- T_331597523_132000_/RConn3 -- bus281/LConn1
  T_122193608_132000_/RConn1 -- L_122193608/LConn1
  T_122193608_132000_/RConn2 -- L_122193608/LConn2
  L_122193608/LConn3 -- T_122193608_132000_/RConn3 -- bus282/LConn1
  T_122112073__/RConn1 -- L_122112073/LConn1
  T_122112073__/RConn2 -- L_122112073/LConn2
  L_122112073/LConn3 -- T_122112073__/RConn3 -- bus283/LConn1
  T_325550726_132000_/RConn1 -- L_325550726/LConn1
  T_325550726_132000_/RConn2 -- L_325550726/LConn2
  L_325550726/LConn3 -- T_325550726_132000_/RConn3 -- bus284/LConn1
  T_119823774_132000_/RConn1 -- L_119823774/LConn1
  T_119823774_132000_/RConn2 -- L_119823774/LConn2
  L_119823774/LConn3 -- T_119823774_132000_/RConn3 -- bus285/LConn1
  T_119823786_132000_/RConn1 -- L_119823786/LConn1
  T_119823786_132000_/RConn2 -- L_119823786/LConn2
  L_119823786/LConn3 -- T_119823786_132000_/RConn3 -- bus286/LConn1
  T_291263083_132000_Tjøme_transformatorstasjon/RConn1 -- L_291263083/LConn1
  T_291263083_132000_Tjøme_transformatorstasjon/RConn2 -- L_291263083/LConn2
  L_291263083/LConn3 -- T_291263083_132000_Tjøme_transformatorstasjon/RConn3 -- bus287/LConn1
  T_291263123_132000_/RConn1 -- L_291263123/LConn1
  T_291263123_132000_/RConn2 -- L_291263123/LConn2
  L_291263123/LConn3 -- T_291263123_132000_/RConn3 -- bus288/LConn1
  T_432917474__/RConn1 -- L_432917474/LConn1
  T_432917474__/RConn2 -- L_432917474/LConn2
  L_432917474/LConn3 -- T_432917474__/RConn3 -- bus289/LConn1
  T_329807471__/RConn1 -- L_329807471/LConn1
  T_329807471__/RConn2 -- L_329807471/LConn2
  L_329807471/LConn3 -- T_329807471__/RConn3 -- bus290/LConn1
  T_329807474__/RConn1 -- L_329807474/LConn1
  T_329807474__/RConn2 -- L_329807474/LConn2
  L_329807474/LConn3 -- T_329807474__/RConn3 -- bus291/LConn1
  T_35602245_132000_/RConn1 -- L_35602245/LConn1
  T_35602245_132000_/RConn2 -- L_35602245/LConn2
  L_35602245/LConn3 -- T_35602245_132000_/RConn3 -- bus292/LConn1
  T_100661361__/RConn1 -- L_100661361/LConn1
  T_100661361__/RConn2 -- L_100661361/LConn2
  L_100661361/LConn3 -- T_100661361__/RConn3 -- bus293/LConn1
  T_100661366_132000_Hauen_transformatorstasjon/RConn1 -- L_100661366/LConn1
  T_100661366_132000_Hauen_transformatorstasjon/RConn2 -- L_100661366/LConn2
  L_100661366/LConn3 -- T_100661366_132000_Hauen_transformatorstasjon/RConn3 -- bus294/LConn1
  T_329807473__/RConn1 -- L_329807473/LConn1
  T_329807473__/RConn2 -- L_329807473/LConn2
  L_329807473/LConn3 -- T_329807473__/RConn3 -- bus295/LConn1
  T_329807476__/RConn1 -- L_329807476/LConn1
  T_329807476__/RConn2 -- L_329807476/LConn2
  L_329807476/LConn3 -- T_329807476__/RConn3 -- bus296/LConn1
  T_100655440_132000_Meen_koblingsstasjon/RConn1 -- L_100655440/LConn1
  T_100655440_132000_Meen_koblingsstasjon/RConn2 -- L_100655440/LConn2
  L_100655440/LConn3 -- T_100655440_132000_Meen_koblingsstasjon/RConn3 -- bus297/LConn1
  T_325545118_132000_/RConn1 -- L_325545118/LConn1
  T_325545118_132000_/RConn2 -- L_325545118/LConn2
  L_325545118/LConn3 -- T_325545118_132000_/RConn3 -- bus298/LConn1
  T_100666299_132000_/RConn1 -- L_100666299/LConn1
  T_100666299_132000_/RConn2 -- L_100666299/LConn2
  L_100666299/LConn3 -- T_100666299_132000_/RConn3 -- bus299/LConn1
  T_329807480_132000_/RConn1 -- L_329807480/LConn1
  T_329807480_132000_/RConn2 -- L_329807480/LConn2
  L_329807480/LConn3 -- T_329807480_132000_/RConn3 -- bus300/LConn1
  T_296272860_132000_/RConn1 -- L_296272860/LConn1
  T_296272860_132000_/RConn2 -- L_296272860/LConn2
  L_296272860/LConn3 -- T_296272860_132000_/RConn3 -- bus301/LConn1
  T_329807483_132000_/RConn1 -- L_329807483/LConn1
  T_329807483_132000_/RConn2 -- L_329807483/LConn2
  L_329807483/LConn3 -- T_329807483_132000_/RConn3 -- bus302/LConn1
  T_120133940__/RConn1 -- L_120133940/LConn1
  T_120133940__/RConn2 -- L_120133940/LConn2
  L_120133940/LConn3 -- T_120133940__/RConn3 -- bus303/LConn1
  T_329581505_132000_/RConn1 -- L_329581505/LConn1
  T_329581505_132000_/RConn2 -- L_329581505/LConn2
  L_329581505/LConn3 -- T_329581505_132000_/RConn3 -- bus304/LConn1
  T_329581506_132000_/RConn1 -- L_329581506/LConn1
  T_329581506_132000_/RConn2 -- L_329581506/LConn2
  L_329581506/LConn3 -- T_329581506_132000_/RConn3 -- bus305/LConn1
  T_329581503_132000_/RConn1 -- L_329581503/LConn1
  T_329581503_132000_/RConn2 -- L_329581503/LConn2
  L_329581503/LConn3 -- T_329581503_132000_/RConn3 -- bus306/LConn1
  T_122234000_132000_/RConn1 -- L_122234000/LConn1
  T_122234000_132000_/RConn2 -- L_122234000/LConn2
  L_122234000/LConn3 -- T_122234000_132000_/RConn3 -- bus307/LConn1
  T_122234005_132000_/RConn1 -- L_122234005/LConn1
  T_122234005_132000_/RConn2 -- L_122234005/LConn2
  L_122234005/LConn3 -- T_122234005_132000_/RConn3 -- bus308/LConn1
  T_122229801_132000_/RConn1 -- L_122229801/LConn1
  T_122229801_132000_/RConn2 -- L_122229801/LConn2
  L_122229801/LConn3 -- T_122229801_132000_/RConn3 -- bus309/LConn1
  T_122228398_132000_/RConn1 -- L_122228398/LConn1
  T_122228398_132000_/RConn2 -- L_122228398/LConn2
  L_122228398/LConn3 -- T_122228398_132000_/RConn3 -- bus310/LConn1
  T_325545116_132000_/RConn1 -- L_325545116/LConn1
  T_325545116_132000_/RConn2 -- L_325545116/LConn2
  L_325545116/LConn3 -- T_325545116_132000_/RConn3 -- bus311/LConn1
  T_108634906__/RConn1 -- L_108634906/LConn1
  T_108634906__/RConn2 -- L_108634906/LConn2
  L_108634906/LConn3 -- T_108634906__/RConn3 -- bus312/LConn1
  T_435669206__/RConn1 -- L_435669206/LConn1
  T_435669206__/RConn2 -- L_435669206/LConn2
  L_435669206/LConn3 -- T_435669206__/RConn3 -- bus313/LConn1
  T_126354422_132000_/RConn1 -- L_126354422/LConn1
  T_126354422_132000_/RConn2 -- L_126354422/LConn2
  L_126354422/LConn3 -- T_126354422_132000_/RConn3 -- bus314/LConn1
  T_100648759_132000_/RConn1 -- L_100648759/LConn1
  T_100648759_132000_/RConn2 -- L_100648759/LConn2
  L_100648759/LConn3 -- T_100648759_132000_/RConn3 -- bus315/LConn1
  T_128985759__/RConn1 -- L_128985759/LConn1
  T_128985759__/RConn2 -- L_128985759/LConn2
  L_128985759/LConn3 -- T_128985759__/RConn3 -- bus316/LConn1
  T_48306065__/RConn1 -- L_48306065/LConn1
  T_48306065__/RConn2 -- L_48306065/LConn2
  L_48306065/LConn3 -- T_48306065__/RConn3 -- bus317/LConn1
  T_50881349__/RConn1 -- L_50881349/LConn1
  T_50881349__/RConn2 -- L_50881349/LConn2
  L_50881349/LConn3 -- T_50881349__/RConn3 -- bus318/LConn1
  T_46832312__/RConn1 -- L_46832312/LConn1
  T_46832312__/RConn2 -- L_46832312/LConn2
  L_46832312/LConn3 -- T_46832312__/RConn3 -- bus319/LConn1
  T_48310010__/RConn1 -- L_48310010/LConn1
  T_48310010__/RConn2 -- L_48310010/LConn2
  L_48310010/LConn3 -- T_48310010__/RConn3 -- bus320/LConn1
  T_107475267_132000_/RConn1 -- L_107475267/LConn1
  T_107475267_132000_/RConn2 -- L_107475267/LConn2
  L_107475267/LConn3 -- T_107475267_132000_/RConn3 -- bus321/LConn1
  T_106966310_132000_/RConn1 -- L_106966310/LConn1
  T_106966310_132000_/RConn2 -- L_106966310/LConn2
  L_106966310/LConn3 -- T_106966310_132000_/RConn3 -- bus322/LConn1
  T_106966308_132000_/RConn1 -- L_106966308/LConn1
  T_106966308_132000_/RConn2 -- L_106966308/LConn2
  L_106966308/LConn3 -- T_106966308_132000_/RConn3 -- bus323/LConn1
  T_29322460_132000_/RConn1 -- L_29322460/LConn1
  T_29322460_132000_/RConn2 -- L_29322460/LConn2
  L_29322460/LConn3 -- T_29322460_132000_/RConn3 -- bus324/LConn1
  T_289829886__/RConn1 -- L_289829886/LConn1
  T_289829886__/RConn2 -- L_289829886/LConn2
  L_289829886/LConn3 -- T_289829886__/RConn3 -- bus325/LConn1
  T_90273576_132000_/RConn1 -- L_90273576/LConn1
  T_90273576_132000_/RConn2 -- L_90273576/LConn2
  L_90273576/LConn3 -- T_90273576_132000_/RConn3 -- bus326/LConn1
  T_90076941_132000_/RConn1 -- L_90076941/LConn1
  T_90076941_132000_/RConn2 -- L_90076941/LConn2
  L_90076941/LConn3 -- T_90076941_132000_/RConn3 -- bus327/LConn1
  T_100651279__/RConn1 -- L_100651279/LConn1
  T_100651279__/RConn2 -- L_100651279/LConn2
  L_100651279/LConn3 -- T_100651279__/RConn3 -- bus328/LConn1
  T_401860888_132000_/RConn1 -- L_401860888/LConn1
  T_401860888_132000_/RConn2 -- L_401860888/LConn2
  L_401860888/LConn3 -- T_401860888_132000_/RConn3 -- bus329/LConn1
  T_100657505_132000_/RConn1 -- L_100657505/LConn1
  T_100657505_132000_/RConn2 -- L_100657505/LConn2
  L_100657505/LConn3 -- T_100657505_132000_/RConn3 -- bus330/LConn1
  T_100677463_132000_/RConn1 -- L_100677463/LConn1
  T_100677463_132000_/RConn2 -- L_100677463/LConn2
  L_100677463/LConn3 -- T_100677463_132000_/RConn3 -- bus331/LConn1
  T_100666317_132000_/RConn1 -- L_100666317/LConn1
  T_100666317_132000_/RConn2 -- L_100666317/LConn2
  L_100666317/LConn3 -- T_100666317_132000_/RConn3 -- bus332/LConn1
  T_296269262__/RConn1 -- L_296269262/LConn1
  T_296269262__/RConn2 -- L_296269262/LConn2
  L_296269262/LConn3 -- T_296269262__/RConn3 -- bus333/LConn1
  T_329581504_132000_/RConn1 -- L_329581504/LConn1
  T_329581504_132000_/RConn2 -- L_329581504/LConn2
  L_329581504/LConn3 -- T_329581504_132000_/RConn3 -- bus334/LConn1
  T_284868564_132000_Øye_sekundærstasjon/RConn1 -- L_284868564/LConn1
  T_284868564_132000_Øye_sekundærstasjon/RConn2 -- L_284868564/LConn2
  L_284868564/LConn3 -- T_284868564_132000_Øye_sekundærstasjon/RConn3 -- bus335/LConn1
  T_285825051__/RConn1 -- L_285825051/LConn1
  T_285825051__/RConn2 -- L_285825051/LConn2
  L_285825051/LConn3 -- T_285825051__/RConn3 -- bus336/LConn1
  T_285915728__/RConn1 -- L_285915728/LConn1
  T_285915728__/RConn2 -- L_285915728/LConn2
  L_285915728/LConn3 -- T_285915728__/RConn3 -- bus337/LConn1
  T_261717967__/RConn1 -- L_261717967/LConn1
  T_261717967__/RConn2 -- L_261717967/LConn2
  L_261717967/LConn3 -- T_261717967__/RConn3 -- bus338/LConn1
  T_128406208__Sylling_trafostasjon/RConn1 -- L_128406208/LConn1
  T_128406208__Sylling_trafostasjon/RConn2 -- L_128406208/LConn2
  L_128406208/LConn3 -- T_128406208__Sylling_trafostasjon/RConn3 -- bus339/LConn1
  T_43078154_300000_Hamang_transformatorstasjon/RConn1 -- L_43078154/LConn1
  T_43078154_300000_Hamang_transformatorstasjon/RConn2 -- L_43078154/LConn2
  L_43078154/LConn3 -- T_43078154_300000_Hamang_transformatorstasjon/RConn3 -- bus340/LConn1
  T_120279477_300000;66000_Minne_transformatorstasjon/RConn1 -- L_120279477/LConn1
  T_120279477_300000;66000_Minne_transformatorstasjon/RConn2 -- L_120279477/LConn2
  L_120279477/LConn3 -- T_120279477_300000;66000_Minne_transformatorstasjon/RConn3 -- bus341/LConn1
  T_113442999_300000_Ulven_trafostasjon/RConn1 -- L_113442999/LConn1
  T_113442999_300000_Ulven_trafostasjon/RConn2 -- L_113442999/LConn2
  L_113442999/LConn3 -- T_113442999_300000_Ulven_trafostasjon/RConn3 -- bus342/LConn1
  T_80179519_300000_/RConn1 -- L_80179519/LConn1
  T_80179519_300000_/RConn2 -- L_80179519/LConn2
  L_80179519/LConn3 -- T_80179519_300000_/RConn3 -- bus343/LConn1
  T_432965765__Blåfalli/RConn1 -- L_432965765/LConn1
  T_432965765__Blåfalli/RConn2 -- L_432965765/LConn2
  L_432965765/LConn3 -- T_432965765__Blåfalli/RConn3 -- bus344/LConn1
  T_285805418_300000_/RConn1 -- L_285805418/LConn1
  T_285805418_300000_/RConn2 -- L_285805418/LConn2
  L_285805418/LConn3 -- T_285805418_300000_/RConn3 -- bus345/LConn1
  T_296078637__/RConn1 -- L_296078637/LConn1
  T_296078637__/RConn2 -- L_296078637/LConn2
  L_296078637/LConn3 -- T_296078637__/RConn3 -- bus346/LConn1
  T_114845318__/RConn1 -- L_114845318/LConn1
  T_114845318__/RConn2 -- L_114845318/LConn2
  L_114845318/LConn3 -- T_114845318__/RConn3 -- bus347/LConn1
  T_114414014_300000_/RConn1 -- L_114414014/LConn1
  T_114414014_300000_/RConn2 -- L_114414014/LConn2
  L_114414014/LConn3 -- T_114414014_300000_/RConn3 -- bus348/LConn1
  T_290562151__/RConn1 -- L_290562151/LConn1
  T_290562151__/RConn2 -- L_290562151/LConn2
  L_290562151/LConn3 -- T_290562151__/RConn3 -- bus349/LConn1
  T_88147266_300000;50000_Stokkeland_trafostasjon/RConn1 -- L_88147266/LConn1
  T_88147266_300000;50000_Stokkeland_trafostasjon/RConn2 -- L_88147266/LConn2
  L_88147266/LConn3 -- T_88147266_300000;50000_Stokkeland_trafostasjon/RConn3 -- bus350/LConn1
  T_46873771_300000_Bærum_trafostasjon/RConn1 -- L_46873771/LConn1
  T_46873771_300000_Bærum_trafostasjon/RConn2 -- L_46873771/LConn2
  L_46873771/LConn3 -- T_46873771_300000_Bærum_trafostasjon/RConn3 -- bus351/LConn1
  T_287115458__/RConn1 -- L_287115458/LConn1
  T_287115458__/RConn2 -- L_287115458/LConn2
  L_287115458/LConn3 -- T_287115458__/RConn3 -- bus352/LConn1
  T_288685602__/RConn1 -- L_288685602/LConn1
  T_288685602__/RConn2 -- L_288685602/LConn2
  L_288685602/LConn3 -- T_288685602__/RConn3 -- bus353/LConn1
  T_284275993_300000_/RConn1 -- L_284275993/LConn1
  T_284275993_300000_/RConn2 -- L_284275993/LConn2
  L_284275993/LConn3 -- T_284275993_300000_/RConn3 -- bus354/LConn1
  T_174418125_300000_Feda_trafostasjon/RConn1 -- L_174418125/LConn1
  T_174418125_300000_Feda_trafostasjon/RConn2 -- L_174418125/LConn2
  L_174418125/LConn3 -- T_174418125_300000_Feda_trafostasjon/RConn3 -- bus355/LConn1
  T_124861857__Kjelland_transformatorstasjon/RConn1 -- L_124861857/LConn1
  T_124861857__Kjelland_transformatorstasjon/RConn2 -- L_124861857/LConn2
  L_124861857/LConn3 -- T_124861857__Kjelland_transformatorstasjon/RConn3 -- bus356/LConn1
  T_295295263__/RConn1 -- L_295295263/LConn1
  T_295295263__/RConn2 -- L_295295263/LConn2
  L_295295263/LConn3 -- T_295295263__/RConn3 -- bus357/LConn1
  T_297392932__Arendal_transformator/RConn1 -- L_297392932/LConn1
  T_297392932__Arendal_transformator/RConn2 -- L_297392932/LConn2
  L_297392932/LConn3 -- T_297392932__Arendal_transformator/RConn3 -- bus358/LConn1
  T_288812256__Songa_kraftverk/RConn1 -- L_288812256/LConn1
  T_288812256__Songa_kraftverk/RConn2 -- L_288812256/LConn2
  L_288812256/LConn3 -- T_288812256__Songa_kraftverk/RConn3 -- bus359/LConn1
  T_265770276__/RConn1 -- L_265770276/LConn1
  T_265770276__/RConn2 -- L_265770276/LConn2
  L_265770276/LConn3 -- T_265770276__/RConn3 -- bus360/LConn1
  T_297388897_300000_Fåberg_trafostasjon/RConn1 -- L_297388897/LConn1
  T_297388897_300000_Fåberg_trafostasjon/RConn2 -- L_297388897/LConn2
  L_297388897/LConn3 -- T_297388897_300000_Fåberg_trafostasjon/RConn3 -- bus361/LConn1
  T_290373414_300000;132000_/RConn1 -- L_290373414/LConn1
  T_290373414_300000;132000_/RConn2 -- L_290373414/LConn2
  L_290373414/LConn3 -- T_290373414_300000;132000_/RConn3 -- bus362/LConn1
  T_290390502_300000_/RConn1 -- L_290390502/LConn1
  T_290390502_300000_/RConn2 -- L_290390502/LConn2
  L_290390502/LConn3 -- T_290390502_300000_/RConn3 -- bus363/LConn1
  T_288810920__/RConn1 -- L_288810920/LConn1
  T_288810920__/RConn2 -- L_288810920/LConn2
  L_288810920/LConn3 -- T_288810920__/RConn3 -- bus364/LConn1
  T_430780474__/RConn1 -- L_430780474/LConn1
  T_430780474__/RConn2 -- L_430780474/LConn2
  L_430780474/LConn3 -- T_430780474__/RConn3 -- bus365/LConn1
  T_285750826__Vinje_kraftverk/RConn1 -- L_285750826/LConn1
  T_285750826__Vinje_kraftverk/RConn2 -- L_285750826/LConn2
  L_285750826/LConn3 -- T_285750826__Vinje_kraftverk/RConn3 -- bus366/LConn1
  T_229396655__/RConn1 -- L_229396655/LConn1
  T_229396655__/RConn2 -- L_229396655/LConn2
  L_229396655/LConn3 -- T_229396655__/RConn3 -- bus367/LConn1
  T_350332649__Samnanger/RConn1 -- L_350332649/LConn1
  T_350332649__Samnanger/RConn2 -- L_350332649/LConn2
  L_350332649/LConn3 -- T_350332649__Samnanger/RConn3 -- bus368/LConn1
  T_289304147__/RConn1 -- L_289304147/LConn1
  T_289304147__/RConn2 -- L_289304147/LConn2
  L_289304147/LConn3 -- T_289304147__/RConn3 -- bus369/LConn1
  T_296076234_300000_/RConn1 -- L_296076234/LConn1
  T_296076234_300000_/RConn2 -- L_296076234/LConn2
  L_296076234/LConn3 -- T_296076234_300000_/RConn3 -- bus370/LConn1
  T_174418126_300000_Feda_static_inverter_plant/RConn1 -- L_174418126/LConn1
  T_174418126_300000_Feda_static_inverter_plant/RConn2 -- L_174418126/LConn2
  L_174418126/LConn3 -- T_174418126_300000_Feda_static_inverter_plant/RConn3 -- bus371/LConn1
  T_400655825_300000;132000_/RConn1 -- L_400655825/LConn1
  T_400655825_300000;132000_/RConn2 -- L_400655825/LConn2
  L_400655825/LConn3 -- T_400655825_300000;132000_/RConn3 -- bus372/LConn1
  T_289304185__/RConn1 -- L_289304185/LConn1
  T_289304185__/RConn2 -- L_289304185/LConn2
  L_289304185/LConn3 -- T_289304185__/RConn3 -- bus373/LConn1
  T_353884513__/RConn1 -- L_353884513/LConn1
  T_353884513__/RConn2 -- L_353884513/LConn2
  L_353884513/LConn3 -- T_353884513__/RConn3 -- bus374/LConn1
  T_242396005__/RConn1 -- L_242396005/LConn1
  T_242396005__/RConn2 -- L_242396005/LConn2
  L_242396005/LConn3 -- T_242396005__/RConn3 -- bus375/LConn1
  T_254428135_300000_/RConn1 -- L_254428135/LConn1
  T_254428135_300000_/RConn2 -- L_254428135/LConn2
  L_254428135/LConn3 -- T_254428135_300000_/RConn3 -- bus376/LConn1
  T_229806969_300000_/RConn1 -- L_229806969/LConn1
  T_229806969_300000_/RConn2 -- L_229806969/LConn2
  L_229806969/LConn3 -- T_229806969_300000_/RConn3 -- bus377/LConn1
  T_229806970__/RConn1 -- L_229806970/LConn1
  T_229806970__/RConn2 -- L_229806970/LConn2
  L_229806970/LConn3 -- T_229806970__/RConn3 -- bus378/LConn1
  T_290393697_420000;300000_Aura/RConn1 -- L_290393697/LConn1
  T_290393697_420000;300000_Aura/RConn2 -- L_290393697/LConn2
  L_290393697/LConn3 -- T_290393697_420000;300000_Aura/RConn3 -- bus379/LConn1
  T_114318083__/RConn1 -- L_114318083/LConn1
  T_114318083__/RConn2 -- L_114318083/LConn2
  L_114318083/LConn3 -- T_114318083__/RConn3 -- bus380/LConn1
  T_114318078__/RConn1 -- L_114318078/LConn1
  T_114318078__/RConn2 -- L_114318078/LConn2
  L_114318078/LConn3 -- T_114318078__/RConn3 -- bus381/LConn1
  T_232893576_420000_Halden/RConn1 -- L_232893576/LConn1
  T_232893576_420000_Halden/RConn2 -- L_232893576/LConn2
  L_232893576/LConn3 -- T_232893576_420000_Halden/RConn3 -- bus382/LConn1
  T_51856017__/RConn1 -- L_51856017/LConn1
  T_51856017__/RConn2 -- L_51856017/LConn2
  L_51856017/LConn3 -- T_51856017__/RConn3 -- bus383/LConn1
  T_51855380__/RConn1 -- L_51855380/LConn1
  T_51855380__/RConn2 -- L_51855380/LConn2
  L_51855380/LConn3 -- T_51855380__/RConn3 -- bus384/LConn1
  T_100151486_420000_Ski/RConn1 -- L_100151486/LConn1
  T_100151486_420000_Ski/RConn2 -- L_100151486/LConn2
  L_100151486/LConn3 -- T_100151486_420000_Ski/RConn3 -- bus385/LConn1
  T_29578389_420000_/RConn1 -- L_29578389/LConn1
  T_29578389_420000_/RConn2 -- L_29578389/LConn2
  L_29578389/LConn3 -- T_29578389_420000_/RConn3 -- bus386/LConn1
  T_206628453__Grenland/RConn1 -- L_206628453/LConn1
  T_206628453__Grenland/RConn2 -- L_206628453/LConn2
  L_206628453/LConn3 -- T_206628453__Grenland/RConn3 -- bus387/LConn1
  T_296238635__/RConn1 -- L_296238635/LConn1
  T_296238635__/RConn2 -- L_296238635/LConn2
  L_296238635/LConn3 -- T_296238635__/RConn3 -- bus388/LConn1
  T_296229069__/RConn1 -- L_296229069/LConn1
  T_296229069__/RConn2 -- L_296229069/LConn2
  L_296229069/LConn3 -- T_296229069__/RConn3 -- bus389/LConn1
  T_197866182_420000;132000_/RConn1 -- L_197866182/LConn1
  T_197866182_420000;132000_/RConn2 -- L_197866182/LConn2
  L_197866182/LConn3 -- T_197866182_420000;132000_/RConn3 -- bus390/LConn1
  T_295444089_420000_Ådal_trafostasjon/RConn1 -- L_295444089/LConn1
  T_295444089_420000_Ådal_trafostasjon/RConn2 -- L_295444089/LConn2
  L_295444089/LConn3 -- T_295444089_420000_Ådal_trafostasjon/RConn3 -- bus391/LConn1
  T_287685850_420000;300000_/RConn1 -- L_287685850/LConn1
  T_287685850_420000;300000_/RConn2 -- L_287685850/LConn2
  L_287685850/LConn3 -- T_287685850_420000;300000_/RConn3 -- bus392/LConn1
  T_287684722_420000_/RConn1 -- L_287684722/LConn1
  T_287684722_420000_/RConn2 -- L_287684722/LConn2
  L_287684722/LConn3 -- T_287684722_420000_/RConn3 -- bus393/LConn1
